simulink model "aocs_plant"  (R2025a)
settings: Solver=ode45  StartTime=0  StopTime=200  RelTol=1e-09  AbsTol=1e-10
undefined symbols (not defined in the file): AOCS, AOCS_Config, AOCS_EnvironmentConfig, AOCS_GNCConfig, AOCS_OrbitConfig, AOCS_SensorConfig, IAU, juliandate, propagateOnboardSgp4
libraries: aerolibtransform2 x8, simulink x8, matrix_library x5
(part 2 of 3)

== system aocs_plant/GNC/Onboard Reference Vectors/Reference Validity ==
  SunVector : Inport
  MagneticVector : Inport  Port=2
  MinimumNorm : Inport  Port=3
  OrbitValid : Inport  Port=4
  Enabled : Inport  Port=5
  Magnetic Exists : RelationalOperator  Operator=>  OutDataTypeStr=boolean  RndMeth=Simplest  InputSameDT=off
  Magnetic Norm Squared : DotProduct  OutDataTypeStr=Inherit: Inherit via internal rule
  Minimum Norm Squared : Product
  References Valid : Logic  Inputs=4  AllPortsSameDT=off  OutDataTypeStr=boolean
  Sun Exists : RelationalOperator  Operator=>  OutDataTypeStr=boolean  RndMeth=Simplest  InputSameDT=off
  Sun Norm Squared : DotProduct  OutDataTypeStr=Inherit: Inherit via internal rule
  To Double : DataTypeConversion  OutDataTypeStr=double  SaturateOnIntegerOverflow=off  RndMeth=Floor
  Valid : Outport
  wires:
  Minimum Norm Squared/1 -> Sun Exists/2, Magnetic Exists/2
  Sun Exists/1 -> References Valid/1
  Magnetic Exists/1 -> References Valid/2
  OrbitValid/1 -> References Valid/3
  Enabled/1 -> References Valid/4
  References Valid/1 -> To Double/1
  To Double/1 -> Valid/1
  SunVector/1 -> Sun Norm Squared/2, Sun Norm Squared/1
  MagneticVector/1 -> Magnetic Norm Squared/2, Magnetic Norm Squared/1
  MinimumNorm/1 -> Minimum Norm Squared/2, Minimum Norm Squared/1
  Sun Norm Squared/1 -> Sun Exists/1
  Magnetic Norm Squared/1 -> Magnetic Exists/1

== system aocs_plant/GNC/Onboard Reference Vectors/Sun Reference Model ==
  r_I_m : Inport
  EnvironmentContext : Inport  Port=2  OutDataTypeStr=Bus: EnvironmentContextBus
  MinimumVectorNorm : Inport  Port=3
  Julian Date : Sum
  Normalize Sun Vector : Subsystem
  Planetary Ephemeris : PlanetaryEphem  units=m,m/s  target=Sun  useDateRange=on  startDate=juliandate(2020, 1, 1, 0, 0, 0)  endDate=juliandate(2030, 1, 1, 0, 0, 0)  outputVelocity=off
  Seconds to Julian Days : Gain  Gain=1/86400
  Select Time Context : BusSelector  OutputSignals=epoch_tdb_jd,t_s
  Spacecraft to Sun Vector : Sum  Inputs=+-
  Sun Vector Column : Reshape  OutputDimensionality=Customize  OutputDimensions=[3 1]
  Unused Sun Distance : Terminator
  sun_I_unit : Outport
  wires:
  EnvironmentContext/1 -> Select Time Context/1
  Select Time Context/2 -> Seconds to Julian Days/1  "<t_s>"
  Select Time Context/1 -> Julian Date/1  "<epoch_tdb_jd>"
  Seconds to Julian Days/1 -> Julian Date/2
  Julian Date/1 -> Planetary Ephemeris/1
  Planetary Ephemeris/1 -> Sun Vector Column/1
  Sun Vector Column/1 -> Spacecraft to Sun Vector/1
  r_I_m/1 -> Spacecraft to Sun Vector/2
  Spacecraft to Sun Vector/1 -> Normalize Sun Vector/1(Vector)
  MinimumVectorNorm/1 -> Normalize Sun Vector/2(MinimumNorm)
  Normalize Sun Vector/1(UnitVector) -> sun_I_unit/1
  Normalize Sun Vector/2(VectorNorm) -> Unused Sun Distance/1

== system aocs_plant/GNC/TRIAD Initialization/CSS Freshness ==
  CurrentTime : Inport
  ReportValid : Inport  Port=2
  ReceiveTime : Inport  Port=3
  Enabled : Inport  Port=4
  MaxAge : Inport  Port=5
  Age Within Limit : RelationalOperator  Operator=<=  OutDataTypeStr=boolean  RndMeth=Simplest  InputSameDT=off
  Fresh : Logic  Inputs=3  AllPortsSameDT=off  OutDataTypeStr=boolean
  Half : Constant  Value=0.5
  Report Age : Sum  Inputs=+-
  Report Is Valid : RelationalOperator  Operator=>  OutDataTypeStr=boolean  RndMeth=Simplest  InputSameDT=off
  Subsystem Enabled : RelationalOperator  Operator=>  OutDataTypeStr=boolean  RndMeth=Simplest  InputSameDT=off
  To Double : DataTypeConversion  OutDataTypeStr=double  SaturateOnIntegerOverflow=off  RndMeth=Floor
  Current : Outport
  wires:
  CurrentTime/1 -> Report Age/1
  ReceiveTime/1 -> Report Age/2
  Report Age/1 -> Age Within Limit/1
  MaxAge/1 -> Age Within Limit/2
  ReportValid/1 -> Report Is Valid/1
  Half/1 -> Report Is Valid/2, Subsystem Enabled/2
  Enabled/1 -> Subsystem Enabled/1
  Age Within Limit/1 -> Fresh/1
  Report Is Valid/1 -> Fresh/2
  Subsystem Enabled/1 -> Fresh/3
  Fresh/1 -> To Double/1
  To Double/1 -> Current/1

== system aocs_plant/GNC/TRIAD Initialization/Magnetometer Freshness ==
  CurrentTime : Inport
  ReportValid : Inport  Port=2
  ReceiveTime : Inport  Port=3
  Enabled : Inport  Port=4
  MaxAge : Inport  Port=5
  Age Within Limit : RelationalOperator  Operator=<=  OutDataTypeStr=boolean  RndMeth=Simplest  InputSameDT=off
  Fresh : Logic  Inputs=3  AllPortsSameDT=off  OutDataTypeStr=boolean
  Half : Constant  Value=0.5
  Report Age : Sum  Inputs=+-
  Report Is Valid : RelationalOperator  Operator=>  OutDataTypeStr=boolean  RndMeth=Simplest  InputSameDT=off
  Subsystem Enabled : RelationalOperator  Operator=>  OutDataTypeStr=boolean  RndMeth=Simplest  InputSameDT=off
  To Double : DataTypeConversion  OutDataTypeStr=double  SaturateOnIntegerOverflow=off  RndMeth=Floor
  Current : Outport
  wires:
  CurrentTime/1 -> Report Age/1
  ReceiveTime/1 -> Report Age/2
  Report Age/1 -> Age Within Limit/1
  MaxAge/1 -> Age Within Limit/2
  ReportValid/1 -> Report Is Valid/1
  Half/1 -> Report Is Valid/2, Subsystem Enabled/2
  Enabled/1 -> Subsystem Enabled/1
  Age Within Limit/1 -> Fresh/1
  Report Is Valid/1 -> Fresh/2
  Subsystem Enabled/1 -> Fresh/3
  Fresh/1 -> To Double/1
  To Double/1 -> Current/1

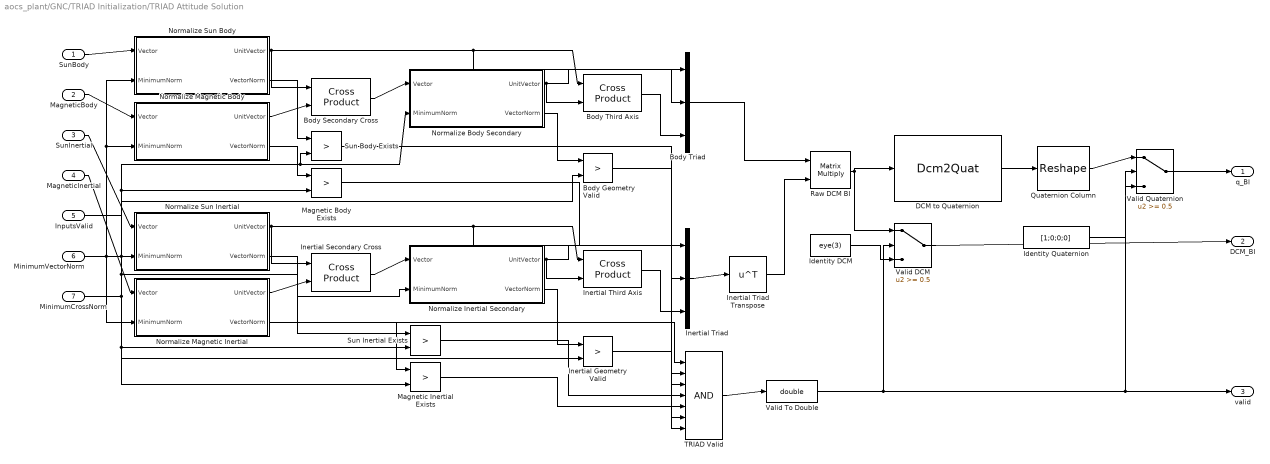
== system aocs_plant/GNC/TRIAD Initialization/TRIAD Attitude Solution ==
  SunBody : Inport
  MagneticBody : Inport  Port=2
  SunInertial : Inport  Port=3
  MagneticInertial : Inport  Port=4
  InputsValid : Inport  Port=5
  MinimumVectorNorm : Inport  Port=6
  MinimumCrossNorm : Inport  Port=7
  Body Geometry Valid : RelationalOperator  Operator=>  OutDataTypeStr=boolean  RndMeth=Simplest  InputSameDT=off
  Body Secondary Cross : matrix_library/Cross Product
  Body Third Axis : matrix_library/Cross Product
  Body Triad : Concatenate  NumInputs=3  Mode=Multidimensional array  ConcatenateDimension=2
  DCM to Quaternion : Dcm2Quat
  Identity DCM : Constant  Value=eye(3)
  Identity Quaternion : Constant  Value=[1;0;0;0]
  Inertial Geometry Valid : RelationalOperator  Operator=>  OutDataTypeStr=boolean  RndMeth=Simplest  InputSameDT=off
  Inertial Secondary Cross : matrix_library/Cross Product
  Inertial Third Axis : matrix_library/Cross Product
  Inertial Triad : Concatenate  NumInputs=3  Mode=Multidimensional array  ConcatenateDimension=2
  Inertial Triad Transpose : Math  Operator=transpose
  Magnetic Body Exists : RelationalOperator  Operator=>  OutDataTypeStr=boolean  RndMeth=Simplest  InputSameDT=off
  Magnetic Inertial Exists : RelationalOperator  Operator=>  OutDataTypeStr=boolean  RndMeth=Simplest  InputSameDT=off
  Normalize Body Secondary : Subsystem
  Normalize Inertial Secondary : Subsystem
  Normalize Magnetic Body : Subsystem
  Normalize Magnetic Inertial : Subsystem
  Normalize Sun Body : Subsystem
  Normalize Sun Inertial : Subsystem
  Quaternion Column : Reshape  OutputDimensionality=Customize  OutputDimensions=[4 1]
  Raw DCM BI : Product  Multiplication=Matrix(*)
  Sun Body Exists : RelationalOperator  Operator=>  OutDataTypeStr=boolean  RndMeth=Simplest  InputSameDT=off
  Sun Inertial Exists : RelationalOperator  Operator=>  OutDataTypeStr=boolean  RndMeth=Simplest  InputSameDT=off
  TRIAD Valid : Logic  Inputs=7  AllPortsSameDT=off  OutDataTypeStr=boolean
  Valid DCM : Switch  Threshold=0.5  SaturateOnIntegerOverflow=off  InputSameDT=off
  Valid Quaternion : Switch  Threshold=0.5  SaturateOnIntegerOverflow=off  InputSameDT=off
  Valid To Double : DataTypeConversion  OutDataTypeStr=double  SaturateOnIntegerOverflow=off  RndMeth=Floor
  q_BI : Outport
  DCM_BI : Outport  Port=2
  valid : Outport  Port=3
  wires:
  SunBody/1 -> Normalize Sun Body/1(Vector)
  MinimumVectorNorm/1 -> Sun Inertial Exists/2, Magnetic Inertial Exists/2, Normalize Inertial Secondary/2(MinimumNorm), Normalize Body Secondary/2(MinimumNorm), Sun Body Exists/2, Magnetic Body Exists/2, Normalize Sun Inertial/2(MinimumNorm), Normalize Sun Body/2(MinimumNorm), Normalize Magnetic Body/2(MinimumNorm), Normalize Magnetic Inertial/2(MinimumNorm)
  MagneticBody/1 -> Normalize Magnetic Body/1(Vector)
  SunInertial/1 -> Normalize Sun Inertial/1(Vector)
  MagneticInertial/1 -> Normalize Magnetic Inertial/1(Vector)
  Normalize Sun Body/1(UnitVector) -> Body Third Axis/1, Body Triad/1, Body Secondary Cross/1
  Normalize Magnetic Body/1(UnitVector) -> Body Secondary Cross/2
  Body Secondary Cross/1 -> Normalize Body Secondary/1(Vector)
  Normalize Body Secondary/1(UnitVector) -> Body Third Axis/2, Body Triad/2
  Body Third Axis/1 -> Body Triad/3
  Normalize Sun Inertial/1(UnitVector) -> Inertial Third Axis/1, Inertial Triad/1, Inertial Secondary Cross/1
  Normalize Magnetic Inertial/1(UnitVector) -> Inertial Secondary Cross/2
  Inertial Secondary Cross/1 -> Normalize Inertial Secondary/1(Vector)
  Normalize Inertial Secondary/1(UnitVector) -> Inertial Third Axis/2, Inertial Triad/2
  Inertial Third Axis/1 -> Inertial Triad/3
  Inertial Triad/1 -> Inertial Triad Transpose/1
  Body Triad/1 -> Raw DCM BI/1
  Inertial Triad Transpose/1 -> Raw DCM BI/2
  Raw DCM BI/1 -> DCM to Quaternion/1, Valid DCM/1
  DCM to Quaternion/1 -> Quaternion Column/1
  Normalize Sun Body/2(VectorNorm) -> Sun Body Exists/1
  Normalize Magnetic Body/2(VectorNorm) -> Magnetic Body Exists/1
  Normalize Sun Inertial/2(VectorNorm) -> Sun Inertial Exists/1
  Normalize Magnetic Inertial/2(VectorNorm) -> Magnetic Inertial Exists/1
  Normalize Body Secondary/2(VectorNorm) -> Body Geometry Valid/1
  MinimumCrossNorm/1 -> Body Geometry Valid/2, Inertial Geometry Valid/2
  Normalize Inertial Secondary/2(VectorNorm) -> Inertial Geometry Valid/1
  InputsValid/1 -> TRIAD Valid/1
  Sun Body Exists/1 -> TRIAD Valid/2
  Magnetic Body Exists/1 -> TRIAD Valid/3
  Sun Inertial Exists/1 -> TRIAD Valid/4
  Magnetic Inertial Exists/1 -> TRIAD Valid/5
  Body Geometry Valid/1 -> TRIAD Valid/6
  Inertial Geometry Valid/1 -> TRIAD Valid/7
  TRIAD Valid/1 -> Valid To Double/1
  Quaternion Column/1 -> Valid Quaternion/1
  Valid To Double/1 -> Valid Quaternion/2, valid/1, Valid DCM/2
  Identity Quaternion/1 -> Valid Quaternion/3
  Identity DCM/1 -> Valid DCM/3
  Valid Quaternion/1 -> q_BI/1
  Valid DCM/1 -> DCM_BI/1

== system aocs_plant/Sensors/GNSS/Fix Availability ==
  GnssConfig : Inport
  Acquisition Complete : RelationalOperator  OutDataTypeStr=boolean  RndMeth=Simplest  InputSameDT=off
  Configured Dropout : simulink/Logic and Bit Operations/Compare To Constant  relop===  const=2  OutDataTypeStr=boolean
  Dropout Uniform : UniformRandomNumber  Minimum=0  Seed=AOCS_SensorConfig.GNSS.dropout_seed  SampleTime=AOCS_SensorConfig.GNSS.sample_time_s
  Fix Available : Logic  Inputs=3  AllPortsSameDT=off  OutDataTypeStr=boolean
  No Configured Dropout : Logic  Operator=NOT  AllPortsSameDT=off  OutDataTypeStr=boolean
  No Random Dropout : Logic  Operator=NOT  AllPortsSameDT=off  OutDataTypeStr=boolean
  Random Dropout : RelationalOperator  Operator=<  OutDataTypeStr=boolean  RndMeth=Simplest  InputSameDT=off
  Select Availability Config : BusSelector  OutputSignals=mode_id,acquisition_time_s,dropout_probability_per_sample
  Simulation Time : Clock
  To Double : DataTypeConversion  OutDataTypeStr=double  SaturateOnIntegerOverflow=off  RndMeth=Floor
  fix_available : Outport
  wires:
  GnssConfig/1 -> Select Availability Config/1
  Simulation Time/1 -> Acquisition Complete/1
  Select Availability Config/2 -> Acquisition Complete/2  "<acquisition_time_s>"
  Dropout Uniform/1 -> Random Dropout/1
  Select Availability Config/3 -> Random Dropout/2  "<dropout_probability_per_sample>"
  Select Availability Config/1 -> Configured Dropout/1  "<mode_id>"
  Random Dropout/1 -> No Random Dropout/1
  Configured Dropout/1 -> No Configured Dropout/1
  Acquisition Complete/1 -> Fix Available/1
  No Random Dropout/1 -> Fix Available/2
  No Configured Dropout/1 -> Fix Available/3
  Fix Available/1 -> To Double/1
  To Double/1 -> fix_available/1  "fix_available"

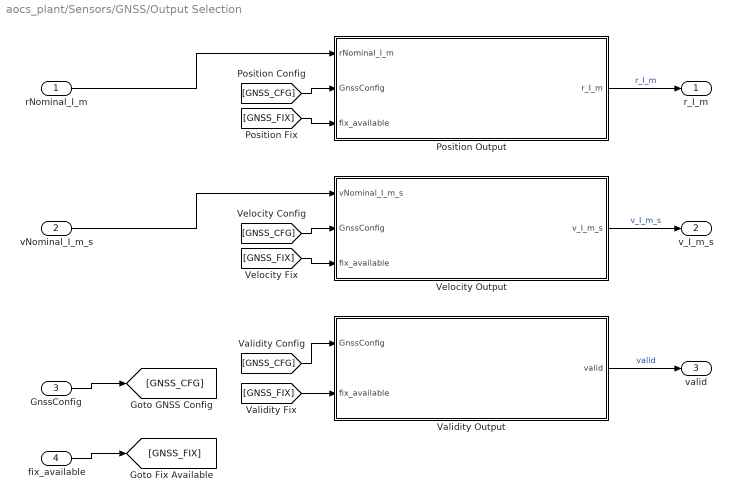
== system aocs_plant/Sensors/GNSS/Output Selection ==
  rNominal_I_m : Inport
  vNominal_I_m_s : Inport  Port=2
  GnssConfig : Inport  Port=3
  fix_available : Inport  Port=4
  Position Output : Subsystem
  Validity Output : Subsystem
  Velocity Output : Subsystem
  r_I_m : Outport
  v_I_m_s : Outport  Port=2
  valid : Outport  Port=3
  wires:
  GnssConfig/1 -> [GNSS_CFG]
  fix_available/1 -> [GNSS_FIX]
  rNominal_I_m/1 -> Position Output/1(rNominal_I_m)
  [GNSS_CFG] -> Position Output/2(GnssConfig)
  [GNSS_FIX] -> Position Output/3(fix_available)
  Position Output/1(r_I_m) -> r_I_m/1  "r_I_m"
  vNominal_I_m_s/1 -> Velocity Output/1(vNominal_I_m_s)
  [GNSS_CFG] -> Velocity Output/2(GnssConfig)
  [GNSS_FIX] -> Velocity Output/3(fix_available)
  Velocity Output/1(v_I_m_s) -> v_I_m_s/1  "v_I_m_s"
  [GNSS_CFG] -> Validity Output/1(GnssConfig)
  [GNSS_FIX] -> Validity Output/2(fix_available)
  Validity Output/1(valid) -> valid/1  "valid"

== system aocs_plant/Sensors/GNSS/PVT Error Model ==
  rTruth_I_m : Inport
  vTruth_I_m_s : Inport  Port=2
  Apply RTN Errors : MATLAB Function  TreatAsAtomicUnit=on
  Position Error RTN : Subsystem
  Velocity Error RTN : Subsystem
  rMeasured_I_m : Outport
  vMeasured_I_m_s : Outport  Port=2
  wires:
  rTruth_I_m/1 -> Apply RTN Errors/1(rTruth_I_m)
  vTruth_I_m_s/1 -> Apply RTN Errors/2(vTruth_I_m_s)
  Position Error RTN/1(positionError_RTN_m) -> Apply RTN Errors/3(positionError_RTN_m)
  Velocity Error RTN/1(velocityError_RTN_m_s) -> Apply RTN Errors/4(velocityError_RTN_m_s)
  Apply RTN Errors/1(rMeasured_I_m) -> rMeasured_I_m/1  "r_measured_I_m"
  Apply RTN Errors/2(vMeasured_I_m_s) -> vMeasured_I_m_s/1  "v_measured_I_m_s"

== system aocs_plant/Sensors/Gyro/Bias ==
  Add : Sum
  Gain : Gain  Gain=AOCS_SensorConfig.Gyro.bias_random_walk_step_std_rad_s
  Random Number : RandomNumber  Seed=AOCS_SensorConfig.Gyro.bias_seed  SampleTime=AOCS_SensorConfig.Gyro.gyro_sample_time_s
  Unit Delay : UnitDelay  InitialCondition=AOCS_SensorConfig.Gyro.bias_initial_rad_s  SampleTime=AOCS_SensorConfig.Gyro.gyro_sample_time_s  HasFrameUpgradeWarning=on
  bias_rad_s : Outport
  wires:
  Random Number/1 -> Gain/1
  Gain/1 -> Add/1
  Add/1 -> Unit Delay/1
  Unit Delay/1 -> Add/2, bias_rad_s/1

== system aocs_plant/Sensors/Magnetometer/Bias ==
  Add : Sum
  Gain : Gain  Gain=AOCS_SensorConfig.Magnetometer.bias_random_walk_step_std_T
  Random Number : RandomNumber  Seed=AOCS_SensorConfig.Magnetometer.bias_seed  SampleTime=AOCS_SensorConfig.Magnetometer.sample_time_s
  Unit Delay : UnitDelay  InitialCondition=AOCS_SensorConfig.Magnetometer.bias_initial_T  SampleTime=AOCS_SensorConfig.Magnetometer.sample_time_s  HasFrameUpgradeWarning=on
  bias_T : Outport
  wires:
  Unit Delay/1 -> bias_T/1, Add/2
  Add/1 -> Unit Delay/1
  Gain/1 -> Add/1
  Random Number/1 -> Gain/1

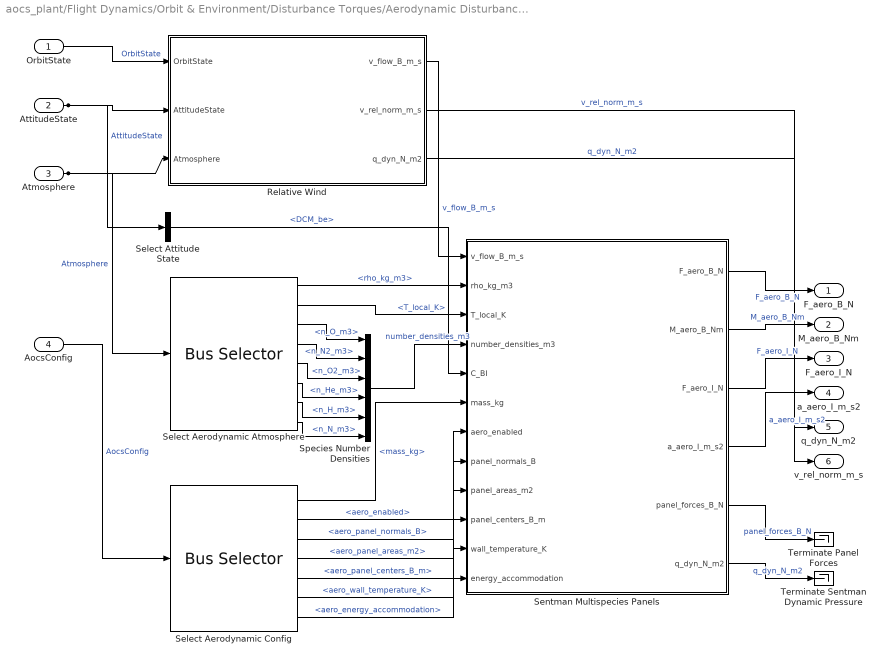
== system aocs_plant/Flight Dynamics/Orbit & Environment/Disturbance Torques/Aerodynamic Disturbance Path ==
  OrbitState : Inport
  AttitudeState : Inport  Port=2
  Atmosphere : Inport  Port=3
  AocsConfig : Inport  Port=4
  Relative Wind : Subsystem
  Select Aerodynamic Atmosphere : BusSelector  OutputSignals=rho_kg_m3,T_local_K,n_O_m3,n_N2_m3,n_O2_m3,n_He_m3,n_H_m3,n_N_m3
  Select Aerodynamic Config : BusSelector  OutputSignals=mass_kg,aero_enabled,aero_panel_normals_B,aero_panel_areas_m2,aero_panel_centers_B_m,aero_wall_temperature_K,aero_energy_accommodation
  Select Attitude State : BusSelector  OutputSignals=DCM_be
  Sentman Multispecies Panels : MATLAB Function  TreatAsAtomicUnit=on
  Species Number Densities : Mux  Inputs=6
  Terminate Panel Forces : Terminator
  Terminate Sentman Dynamic Pressure : Terminator
  F_aero_B_N : Outport
  M_aero_B_Nm : Outport  Port=2
  F_aero_I_N : Outport  Port=3
  a_aero_I_m_s2 : Outport  Port=4
  q_dyn_N_m2 : Outport  Port=5
  v_rel_norm_m_s : Outport  Port=6
  wires:
  OrbitState/1 -> Relative Wind/1(OrbitState)  "OrbitState"
  AttitudeState/1 -> Relative Wind/2(AttitudeState), Select Attitude State/1  "AttitudeState"
  Atmosphere/1 -> Relative Wind/3(Atmosphere), Select Aerodynamic Atmosphere/1  "Atmosphere"
  AocsConfig/1 -> Select Aerodynamic Config/1  "AocsConfig"
  Relative Wind/1(v_flow_B_m_s) -> Sentman Multispecies Panels/1(v_flow_B_m_s)  "v_flow_B_m_s"
  Select Aerodynamic Atmosphere/1 -> Sentman Multispecies Panels/2(rho_kg_m3)  "<rho_kg_m3>"
  Select Aerodynamic Atmosphere/2 -> Sentman Multispecies Panels/3(T_local_K)  "<T_local_K>"
  Select Aerodynamic Atmosphere/3 -> Species Number Densities/1  "<n_O_m3>"
  Select Aerodynamic Atmosphere/4 -> Species Number Densities/2  "<n_N2_m3>"
  Select Aerodynamic Atmosphere/5 -> Species Number Densities/3  "<n_O2_m3>"
  Select Aerodynamic Atmosphere/6 -> Species Number Densities/4  "<n_He_m3>"
  Select Aerodynamic Atmosphere/7 -> Species Number Densities/5  "<n_H_m3>"
  Select Aerodynamic Atmosphere/8 -> Species Number Densities/6  "<n_N_m3>"
  Species Number Densities/1 -> Sentman Multispecies Panels/4(number_densities_m3)  "number_densities_m3"
  Select Attitude State/1 -> Sentman Multispecies Panels/5(C_BI)  "<DCM_be>"
  Select Aerodynamic Config/1 -> Sentman Multispecies Panels/6(mass_kg)  "<mass_kg>"
  Select Aerodynamic Config/2 -> Sentman Multispecies Panels/7(aero_enabled)  "<aero_enabled>"
  Select Aerodynamic Config/3 -> Sentman Multispecies Panels/8(panel_normals_B)  "<aero_panel_normals_B>"
  Select Aerodynamic Config/4 -> Sentman Multispecies Panels/9(panel_areas_m2)  "<aero_panel_areas_m2>"
  Select Aerodynamic Config/5 -> Sentman Multispecies Panels/10(panel_centers_B_m)  "<aero_panel_centers_B_m>"
  Select Aerodynamic Config/6 -> Sentman Multispecies Panels/11(wall_temperature_K)  "<aero_wall_temperature_K>"
  Select Aerodynamic Config/7 -> Sentman Multispecies Panels/12(energy_accommodation)  "<aero_energy_accommodation>"
  Sentman Multispecies Panels/1(F_aero_B_N) -> F_aero_B_N/1  "F_aero_B_N"
  Sentman Multispecies Panels/2(M_aero_B_Nm) -> M_aero_B_Nm/1  "M_aero_B_Nm"
  Sentman Multispecies Panels/3(F_aero_I_N) -> F_aero_I_N/1  "F_aero_I_N"
  Sentman Multispecies Panels/4(a_aero_I_m_s2) -> a_aero_I_m_s2/1  "a_aero_I_m_s2"
  Relative Wind/3(q_dyn_N_m2) -> q_dyn_N_m2/1  "q_dyn_N_m2"
  Relative Wind/2(v_rel_norm_m_s) -> v_rel_norm_m_s/1  "v_rel_norm_m_s"
  Sentman Multispecies Panels/5(panel_forces_B_N) -> Terminate Panel Forces/1  "panel_forces_B_N"
  Sentman Multispecies Panels/6(q_dyn_N_m2) -> Terminate Sentman Dynamic Pressure/1  "q_dyn_N_m2"

== system aocs_plant/Flight Dynamics/Orbit & Environment/Disturbance Torques/Gravity Gradient Path ==
  OrbitState : Inport
  AttitudeState : Inport  Port=2
  AocsConfig : Inport  Port=3
  EnvironmentContext : Inport  Port=4
  EnvironmentConfig : Inport  Port=5
  Apply GG Enable : Product
  Gravity Gradient Torque : MATLAB Function  TreatAsAtomicUnit=on
  Select AOCS Config : BusSelector  OutputSignals=I_B
  Select Attitude State : BusSelector  OutputSignals=DCM_be
  Select Environment Config : BusSelector  OutputSignals=gravity_gradient_enabled
  Select Environment Context : BusSelector  OutputSignals=mu_m3_s2
  Select Orbit State : BusSelector  OutputSignals=r_I_m
  M_gg_B_Nm : Outport
  wires:
  OrbitState/1 -> Select Orbit State/1  "OrbitState"
  AttitudeState/1 -> Select Attitude State/1  "AttitudeState"
  AocsConfig/1 -> Select AOCS Config/1  "AocsConfig"
  EnvironmentContext/1 -> Select Environment Context/1  "EnvironmentContext"
  EnvironmentConfig/1 -> Select Environment Config/1  "EnvironmentConfig"
  Select Orbit State/1 -> Gravity Gradient Torque/1(r_I_m)  "<r_I_m>"
  Select Attitude State/1 -> Gravity Gradient Torque/2(DCM_be)  "<DCM_be>"
  Select AOCS Config/1 -> Gravity Gradient Torque/3(I_B)  "<I_B>"
  Select Environment Context/1 -> Apply GG Enable/1  "<mu_m3_s2>"
  Select Environment Config/1 -> Apply GG Enable/2  "<gravity_gradient_enabled>"
  Apply GG Enable/1 -> Gravity Gradient Torque/4(mu_m3_s2)  "mu_m3_s2"
  Gravity Gradient Torque/1(M_gg_B_Nm) -> M_gg_B_Nm/1  "M_gg_B_Nm"

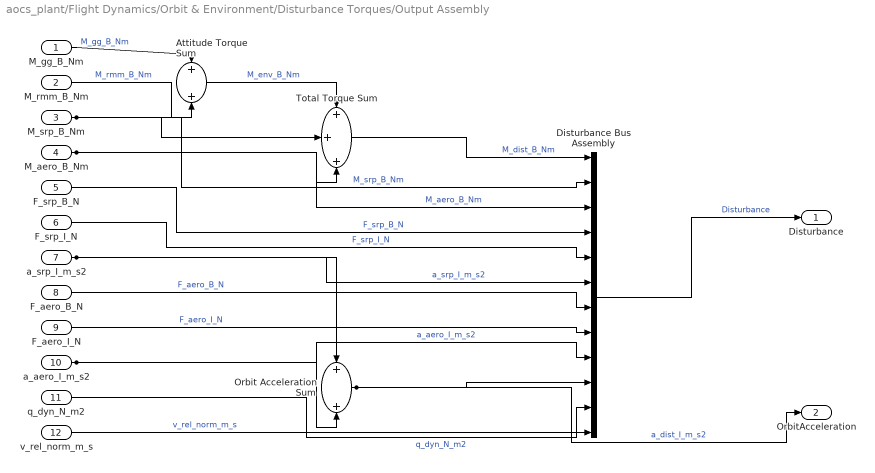
== system aocs_plant/Flight Dynamics/Orbit & Environment/Disturbance Torques/Output Assembly ==
  M_gg_B_Nm : Inport
  M_rmm_B_Nm : Inport  Port=2
  M_srp_B_Nm : Inport  Port=3
  M_aero_B_Nm : Inport  Port=4
  F_srp_B_N : Inport  Port=5
  F_srp_I_N : Inport  Port=6
  a_srp_I_m_s2 : Inport  Port=7
  F_aero_B_N : Inport  Port=8
  F_aero_I_N : Inport  Port=9
  a_aero_I_m_s2 : Inport  Port=10
  q_dyn_N_m2 : Inport  Port=11
  v_rel_norm_m_s : Inport  Port=12
  Attitude Torque Sum : Sum
  Disturbance Bus Assembly : BusCreator  Inputs=12  OutDataTypeStr=Bus: DisturbanceBus
  Orbit Acceleration Sum : Sum
  Total Torque Sum : Sum  Inputs=+++
  Disturbance : Outport
  OrbitAcceleration : Outport  Port=2
  wires:
  M_gg_B_Nm/1 -> Attitude Torque Sum/1  "M_gg_B_Nm"
  M_rmm_B_Nm/1 -> Attitude Torque Sum/2  "M_rmm_B_Nm"
  Attitude Torque Sum/1 -> Total Torque Sum/1  "M_env_B_Nm"
  M_srp_B_Nm/1 -> Total Torque Sum/2, Disturbance Bus Assembly/2  "M_srp_B_Nm"
  M_aero_B_Nm/1 -> Total Torque Sum/3, Disturbance Bus Assembly/3  "M_aero_B_Nm"
  a_srp_I_m_s2/1 -> Orbit Acceleration Sum/1, Disturbance Bus Assembly/6  "a_srp_I_m_s2"
  a_aero_I_m_s2/1 -> Orbit Acceleration Sum/2, Disturbance Bus Assembly/9  "a_aero_I_m_s2"
  Total Torque Sum/1 -> Disturbance Bus Assembly/1  "M_dist_B_Nm"
  F_srp_B_N/1 -> Disturbance Bus Assembly/4  "F_srp_B_N"
  F_srp_I_N/1 -> Disturbance Bus Assembly/5  "F_srp_I_N"
  F_aero_B_N/1 -> Disturbance Bus Assembly/7  "F_aero_B_N"
  F_aero_I_N/1 -> Disturbance Bus Assembly/8  "F_aero_I_N"
  Orbit Acceleration Sum/1 -> Disturbance Bus Assembly/10, OrbitAcceleration/1  "a_dist_I_m_s2"
  q_dyn_N_m2/1 -> Disturbance Bus Assembly/11  "q_dyn_N_m2"
  v_rel_norm_m_s/1 -> Disturbance Bus Assembly/12  "v_rel_norm_m_s"
  Disturbance Bus Assembly/1 -> Disturbance/1  "Disturbance"

== system aocs_plant/Flight Dynamics/Orbit & Environment/Disturbance Torques/Residual Magnetic Path ==
  EnvironmentConfig : Inport
  MagneticField : Inport  Port=2
  Apply RMM Enable : Product
  Cross Product : matrix_library/Cross Product
  Select Environment Config : BusSelector  OutputSignals=m_res_B_A_m2,rmm_enabled
  Select Magnetic Field : BusSelector  OutputSignals=B_B_T
  M_rmm_B_Nm : Outport
  wires:
  EnvironmentConfig/1 -> Select Environment Config/1  "EnvironmentConfig"
  MagneticField/1 -> Select Magnetic Field/1  "MagneticField"
  Select Environment Config/1 -> Apply RMM Enable/1  "<m_res_B_A_m2>"
  Select Environment Config/2 -> Apply RMM Enable/2  "<rmm_enabled>"
  Apply RMM Enable/1 -> Cross Product/1  "m_res_B_A_m2"
  Select Magnetic Field/1 -> Cross Product/2  "<B_B_T>"
  Cross Product/1 -> M_rmm_B_Nm/1  "M_rmm_B_Nm"

== system aocs_plant/Flight Dynamics/Orbit & Environment/Disturbance Torques/SRP Disturbance Path ==
  SRP : Inport
  AttitudeState : Inport  Port=2
  AocsConfig : Inport  Port=3
  SRP Inertial Acceleration : MATLAB Function  TreatAsAtomicUnit=on
  Select Attitude State : BusSelector  OutputSignals=DCM_be
  Select Mass : BusSelector  OutputSignals=mass_kg
  Select SRP : BusSelector  OutputSignals=M_srp_B_Nm,F_srp_B_N
  M_srp_B_Nm : Outport
  F_srp_B_N : Outport  Port=2
  F_srp_I_N : Outport  Port=3
  a_srp_I_m_s2 : Outport  Port=4
  wires:
  SRP/1 -> Select SRP/1  "SRP"
  AttitudeState/1 -> Select Attitude State/1  "AttitudeState"
  AocsConfig/1 -> Select Mass/1  "AocsConfig"
  Select SRP/1 -> M_srp_B_Nm/1  "<M_srp_B_Nm>"
  Select SRP/2 -> SRP Inertial Acceleration/1(F_srp_B_N), F_srp_B_N/1  "<F_srp_B_N>"
  Select Attitude State/1 -> SRP Inertial Acceleration/2(C_BI)  "<DCM_be>"
  Select Mass/1 -> SRP Inertial Acceleration/3(mass_kg)  "<mass_kg>"
  SRP Inertial Acceleration/1(F_srp_I_N) -> F_srp_I_N/1  "F_srp_I_N"
  SRP Inertial Acceleration/2(a_srp_I_m_s2) -> a_srp_I_m_s2/1  "a_srp_I_m_s2"

== system aocs_plant/Flight Dynamics/Orbit & Environment/Environment Products/Atmosphere Products ==
  EnvironmentConfig : Inport  OutDataTypeStr=Bus: EnvironmentConfigBus
  OrbitState : Inport  Port=2  OutDataTypeStr=Bus: OrbitStateBus
  EnvironmentContext : Inport  Port=3  OutDataTypeStr=Bus: EnvironmentContextBus
  Atmosphere Model : Subsystem
  Frame Transformations : Subsystem
  Terminate C_ECEF_ECI : Terminator
  Terminate v_ECEF_m_s : Terminator
  Atmosphere : Outport  OutDataTypeStr=Bus: AtmosphereBus
  wires:
  OrbitState/1 -> Frame Transformations/1(In1), Atmosphere Model/2(OrbitState)
  EnvironmentContext/1 -> Frame Transformations/2(In2), Atmosphere Model/4(EnvironmentContext)
  EnvironmentConfig/1 -> Atmosphere Model/1(EnvironmentConfig)
  Frame Transformations/1(lla) -> Atmosphere Model/3(lla)
  Frame Transformations/2(v_ECEF_m_s) -> Terminate v_ECEF_m_s/1
  Frame Transformations/3(C_ECEF_ECI) -> Terminate C_ECEF_ECI/1
  Atmosphere Model/1(Atmosphere) -> Atmosphere/1

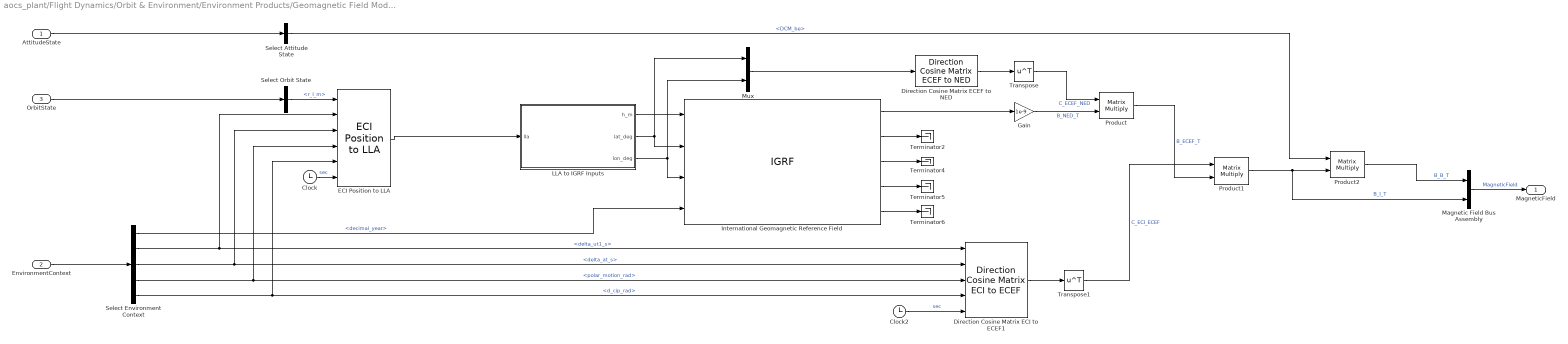
== system aocs_plant/Flight Dynamics/Orbit & Environment/Environment Products/Geomagnetic Field Model ==
  AttitudeState : Inport
  EnvironmentContext : Inport  Port=2
  OrbitState : Inport  Port=3
  Clock : Clock
  Clock2 : Clock
  Direction Cosine Matrix ECEF to NED : aerolibtransform2/Direction Cosine Matrix ECEF to NED
  Direction Cosine Matrix ECI to ECEF1 : aerolibtransform2/Direction Cosine Matrix ECI to ECEF  red=IAU-2000/2006  year=2026  month=January  day=1  hour=0  min=0  sec=0  deltaT=Sec  errorflag=Error  extraparamflag=on
      settings: AttributesFormatString=%<red>
  ECI Position to LLA : aerolibtransform2/ECI Position to LLA  red=IAU-2000/2006  year=2026  month=January  day=1  hour=0  min=0  sec=0  deltaT=Sec  errorflag=Error  extraparamflag=on  eunits=Metric (MKS)  earthmodel=WGS84  flat=1/298.257223563  eqradius=6378137
      settings: AttributesFormatString=%<red>
  Gain : Gain  Gain=1e-9
  International Geomagnetic Reference Field : IGRF  month=January  day=1  sv_out=off
      settings: AttributesFormatString=%<generation>
  LLA to IGRF Inputs : MATLAB Function  TreatAsAtomicUnit=on
  Magnetic Field Bus Assembly : BusCreator  Inputs=2  OutDataTypeStr=Bus: MagneticFieldBus
  Mux : Mux  Inputs=2
  Product : Product  Multiplication=Matrix(*)
  Product1 : Product  Multiplication=Matrix(*)
  Product2 : Product  Multiplication=Matrix(*)
  Select Attitude State : BusSelector  OutputSignals=DCM_be
  Select Environment Context : BusSelector  OutputSignals=decimal_year,delta_ut1_s,delta_at_s,polar_motion_rad,d_cip_rad
  Select Orbit State : BusSelector  OutputSignals=r_I_m
  Terminator{2,4..6} (4 alike) : Terminator
  Transpose : Math  Operator=transpose
  Transpose1 : Math  Operator=transpose
  MagneticField : Outport
  wires:
  Product2/1 -> Magnetic Field Bus Assembly/1  "B_B_T"
  Product1/1 -> Magnetic Field Bus Assembly/2, Product2/2  "B_I_T"
  Transpose1/1 -> Product1/1  "C_ECI_ECEF"
  Product/1 -> Product1/2  "B_ECEF_T"
  Direction Cosine Matrix ECI to ECEF1/1 -> Transpose1/1
  Transpose/1 -> Product/1  "C_ECEF_NED"
  Gain/1 -> Product/2  "B_NED_T"
  Direction Cosine Matrix ECEF to NED/1 -> Transpose/1
  International Geomagnetic Reference Field/2 -> Terminator2/1
  International Geomagnetic Reference Field/1 -> Gain/1
  Mux/1 -> Direction Cosine Matrix ECEF to NED/1
  International Geomagnetic Reference Field/5 -> Terminator6/1
  LLA to IGRF Inputs/2(lat_deg) -> International Geomagnetic Reference Field/2, Mux/1
  International Geomagnetic Reference Field/4 -> Terminator5/1
  LLA to IGRF Inputs/1(h_m) -> International Geomagnetic Reference Field/1
  LLA to IGRF Inputs/3(lon_deg) -> International Geomagnetic Reference Field/3, Mux/2
  International Geomagnetic Reference Field/3 -> Terminator4/1
  ECI Position to LLA/1 -> LLA to IGRF Inputs/1(lla)
  AttitudeState/1 -> Select Attitude State/1
  Select Attitude State/1 -> Product2/1  "<DCM_be>"
  OrbitState/1 -> Select Orbit State/1
  Select Orbit State/1 -> ECI Position to LLA/1  "<r_I_m>"
  EnvironmentContext/1 -> Select Environment Context/1
  Select Environment Context/1 -> International Geomagnetic Reference Field/4  "<decimal_year>"
  Magnetic Field Bus Assembly/1 -> MagneticField/1  "MagneticField"
  Select Environment Context/5 -> ECI Position to LLA/5, Direction Cosine Matrix ECI to ECEF1/4  "<d_cip_rad>"
  Clock/1 -> ECI Position to LLA/6  "sec"
  Clock2/1 -> Direction Cosine Matrix ECI to ECEF1/5  "sec"
  Select Environment Context/4 -> ECI Position to LLA/4, Direction Cosine Matrix ECI to ECEF1/3  "<polar_motion_rad>"
  Select Environment Context/2 -> Direction Cosine Matrix ECI to ECEF1/1, ECI Position to LLA/2  "<delta_ut1_s>"
  Select Environment Context/3 -> ECI Position to LLA/3, Direction Cosine Matrix ECI to ECEF1/2  "<delta_at_s>"

== system aocs_plant/Flight Dynamics/Orbit & Environment/Environment Products/Illumination Model ==
  OrbitState : Inport
  EnvironmentConfig : Inport  Port=2
  Sun : Inport  Port=3
  Eclipse Disabled Visibility : Constant  Value=1.0
  Eclipse Enable Switch : Switch  Threshold=0.5  SaturateOnIntegerOverflow=off  InputSameDT=off
  Eclipse Shadow Model (Dual Cone) : EclipseShadowModel  outputShadowRegion=on  startDate=juliandate(2026, 1, 1, 0, 0, 0)  customRadius=6378137  ephemerisStartDate=juliandate(2020, 1, 1, 0, 0, 0)  ephemerisEndDate=juliandate(2030, 1, 1, 0, 0, 0)
  Illumination Bus Assembly : BusCreator  Inputs=3  OutDataTypeStr=Bus: IlluminationBus
  Select Environment Config : BusSelector  OutputSignals=eclipse_enabled
  Select Orbit State : BusSelector  OutputSignals=r_I_m
  Select Sun : BusSelector  OutputSignals=solar_flux_W_m2
  Solar Flux Shadowing : Product
  Terminator : Terminator
  Terminator1 : Terminator
  Illumination : Outport
  wires:
  Eclipse Shadow Model (Dual Cone)/2 -> Terminator/1
  Eclipse Shadow Model (Dual Cone)/3 -> Terminator1/1
  Eclipse Shadow Model (Dual Cone)/1 -> Illumination Bus Assembly/1, Eclipse Enable Switch/1  "eclipse_fraction"
  OrbitState/1 -> Select Orbit State/1
  Select Orbit State/1 -> Eclipse Shadow Model (Dual Cone)/1  "<r_I_m>"
  EnvironmentConfig/1 -> Select Environment Config/1
  Select Environment Config/1 -> Eclipse Enable Switch/2  "<eclipse_enabled>"
  Eclipse Disabled Visibility/1 -> Eclipse Enable Switch/3
  Sun/1 -> Select Sun/1
  Select Sun/1 -> Solar Flux Shadowing/1  "<solar_flux_W_m2>"
  Eclipse Enable Switch/1 -> Solar Flux Shadowing/2, Illumination Bus Assembly/2  "sun_visibility"
  Solar Flux Shadowing/1 -> Illumination Bus Assembly/3  "solar_flux_shadowed_W_m2"
  Illumination Bus Assembly/1 -> Illumination/1  "Illumination"

== system aocs_plant/Flight Dynamics/Orbit & Environment/Environment Products/Solar Radiation Pressure ==
  Illumination : Inport
  Sun : Inport  Port=2
  MATLAB Function : MATLAB Function  TreatAsAtomicUnit=on
  SRP Bus Assembly : BusCreator  Inputs=3  OutDataTypeStr=Bus: SrpBus
  Select Illumination : BusSelector  OutputSignals=solar_flux_shadowed_W_m2
  Select Sun : BusSelector  OutputSignals=sun_B_unit
  srp_area_ref_m2 : Constant  Value=AOCS.EnvironmentConfig.srp_area_ref_m2  VectorParams1D=off  OutDataTypeStr=double
  srp_center_of_pressure_B_m : Constant  Value=AOCS.EnvironmentConfig.srp_center_of_pressure_B_m  VectorParams1D=off  OutDataTypeStr=double
  srp_coefficient_reflectivity : Constant  Value=AOCS.EnvironmentConfig.srp_coefficient_reflectivity  VectorParams1D=off  OutDataTypeStr=double
  srp_enabled : Constant  Value=AOCS.EnvironmentConfig.srp_enabled  VectorParams1D=off  OutDataTypeStr=double
  SRP : Outport
  wires:
  srp_enabled/1 -> MATLAB Function/3(srp_enabled)
  srp_area_ref_m2/1 -> MATLAB Function/4(srp_area_ref_m2)
  srp_coefficient_reflectivity/1 -> MATLAB Function/5(srp_coefficient_reflectivity)
  srp_center_of_pressure_B_m/1 -> MATLAB Function/6(srp_center_of_pressure_B_m)
  MATLAB Function/2(F_srp_B_N) -> SRP Bus Assembly/2  "F_srp_B_N"
  MATLAB Function/3(P_srp_N_m2) -> SRP Bus Assembly/3  "P_srp_N_m2"
  Sun/1 -> Select Sun/1  "Sun"
  Select Sun/1 -> MATLAB Function/1(sun_B_unit)  "<sun_B_unit>"
  Illumination/1 -> Select Illumination/1  "Illumination"
  Select Illumination/1 -> MATLAB Function/2(solar_flux_shadowed_W_m2)  "<solar_flux_shadowed_W_m2>"
  SRP Bus Assembly/1 -> SRP/1  "SRP"
  MATLAB Function/1(M_srp_B_Nm) -> SRP Bus Assembly/1  "M_srp_B_Nm"

== system aocs_plant/Flight Dynamics/Orbit & Environment/Environment Products/Sun Products ==
  EnvironmentConfig : Inport
  OrbitState : Inport  Port=2
  AttitudeState : Inport  Port=3
  EnvironmentContext : Inport  Port=4
  "  " : BusSelector  OutputSignals=solar_constant_W_m2
  Bus Selector : BusSelector  OutputSignals=r_I_m
  Bus Selector1 : BusSelector  OutputSignals=DCM_be
  Julian Date : Sum
  Planetary Ephemeris : PlanetaryEphem  units=m,m/s  target=Sun  useDateRange=on  startDate=juliandate(2020, 1, 1, 0, 0, 0)  endDate=juliandate(2030, 1, 1, 0, 0, 0)  outputVelocity=off
  Seconds to Julian Days : Gain  Gain=1/86400
  Select Environment Context : BusSelector  OutputSignals=epoch_tdb_jd,t_s
  Sun Bus Assembly : BusCreator  Inputs=5  OutDataTypeStr=Bus: SunBus
  Sun Geometry : MATLAB Function  TreatAsAtomicUnit=on
  Sun Vector Column : Reshape  OutputDimensionality=Customize  OutputDimensions=[3 1]
  Sun : Outport
  wires:
  EnvironmentContext/1 -> Select Environment Context/1
  Seconds to Julian Days/1 -> Julian Date/2
  Julian Date/1 -> Planetary Ephemeris/1
  Sun Geometry/1(sun_B_unit) -> Sun Bus Assembly/1  "sun_B_unit"
  Sun Geometry/2(sun_I_unit) -> Sun Bus Assembly/2  "sun_I_unit"
  Sun Geometry/3(r_sun_I_m) -> Sun Bus Assembly/3  "r_sun_I_m"
  Sun Geometry/4(sun_distance_m) -> Sun Bus Assembly/4  "sun_distance_m"
  Sun Geometry/5(solar_flux_W_m2) -> Sun Bus Assembly/5  "solar_flux_W_m2"
  Planetary Ephemeris/1 -> Sun Vector Column/1
  Sun Vector Column/1 -> Sun Geometry/1(r_sun_I_m_ephem)
  Select Environment Context/2 -> Seconds to Julian Days/1  "<t_s>"
  Select Environment Context/1 -> Julian Date/1  "<epoch_tdb_jd>"
  EnvironmentConfig/1 -> "  "/1
  "  "/1 -> Sun Geometry/2(solar_constant_W_m2)  "<solar_constant_W_m2>"
  OrbitState/1 -> Bus Selector/1
  Bus Selector/1 -> Sun Geometry/3(r_I_m)  "<r_I_m>"
  AttitudeState/1 -> Bus Selector1/1
  Bus Selector1/1 -> Sun Geometry/4(DCM_be)  "<DCM_be>"
  Sun Bus Assembly/1 -> Sun/1  "Sun"

== system aocs_plant/Flight Dynamics/Orbit & Environment/Orbit Propagator & Time/Orbit State ==
  OrbitAcceleration : Inport
  Orbit Propagator : Subsystem
  OrbitState : Outport
  wires:
  Orbit Propagator/1(OrbitState) -> OrbitState/1
  OrbitAcceleration/1 -> Orbit Propagator/1(OrbitAcceleration)

== system aocs_plant/Flight Dynamics/Orbit & Environment/Orbit Propagator & Time/Orbit and Time Context ==
  In1 : Inport
  Clock1 : Clock
  Delta AT : Constant  Value=AOCS.Environment.EarthOrientation.DeltaAT_s  OutDataTypeStr=double
  Delta CIP : Constant  Value=AOCS.Environment.EarthOrientation.DCIP_rad  OutDataTypeStr=double
  Delta UT1 : Constant  Value=AOCS.Environment.EarthOrientation.DeltaUT1_s  OutDataTypeStr=double
  Environment Context Bus Assembly : BusCreator  Inputs=9  OutDataTypeStr=Bus: EnvironmentContextBus
  MATLAB Function : MATLAB Function  TreatAsAtomicUnit=on
  Polar Motion : Constant  Value=AOCS.Environment.EarthOrientation.PolarMotion_rad  OutDataTypeStr=double
  Select Orbit Config : BusSelector  OutputSignals=epoch_utc,mu_m3_s2,epoch_tdb_jd
  EnvironmentContext : Outport
  wires:
  Select Orbit Config/2 -> Environment Context Bus Assembly/2  "<mu_m3_s2>"
  MATLAB Function/1(dyear) -> Environment Context Bus Assembly/1  "decimal_year"
  In1/1 -> Select Orbit Config/1
  Clock1/1 -> Environment Context Bus Assembly/4, MATLAB Function/2(t_s)  "t_s"
  Select Orbit Config/3 -> Environment Context Bus Assembly/5  "<epoch_tdb_jd>"
  Environment Context Bus Assembly/1 -> EnvironmentContext/1  "EnvironmentContext"
  Select Orbit Config/1 -> MATLAB Function/1(epoch_utc), Environment Context Bus Assembly/3  "<epoch_utc>"
  Delta AT/1 -> Environment Context Bus Assembly/6  "delta_at_s"
  Delta UT1/1 -> Environment Context Bus Assembly/7  "delta_ut1_s"
  Polar Motion/1 -> Environment Context Bus Assembly/8  "polar_motion_rad"
  Delta CIP/1 -> Environment Context Bus Assembly/9  "d_cip_rad"

== system aocs_plant/GNC/Onboard Reference Vectors/Sun Reference Model/Normalize Sun Vector ==
  Vector : Inport
  MinimumNorm : Inport  Port=2
  Norm : Math  Operator=sqrt
  Norm Squared : DotProduct  OutDataTypeStr=Inherit: Inherit via internal rule
  Normalize : Product  Inputs=*/
  Safe Norm : MinMax  Function=max  Inputs=2
  UnitVector : Outport
  VectorNorm : Outport  Port=2
  wires:
  Vector/1 -> Normalize/1, Norm Squared/1, Norm Squared/2
  Norm Squared/1 -> Norm/1
  Norm/1 -> VectorNorm/1, Safe Norm/1
  MinimumNorm/1 -> Safe Norm/2
  Safe Norm/1 -> Normalize/2
  Normalize/1 -> UnitVector/1

== system aocs_plant/GNC/TRIAD Initialization/TRIAD Attitude Solution/Normalize Body Secondary ==
  Vector : Inport
  MinimumNorm : Inport  Port=2
  Norm : Math  Operator=sqrt
  Norm Squared : DotProduct  OutDataTypeStr=Inherit: Inherit via internal rule
  Normalize : Product  Inputs=*/
  Safe Norm : MinMax  Function=max  Inputs=2
  UnitVector : Outport
  VectorNorm : Outport  Port=2
  wires:
  Vector/1 -> Norm Squared/1, Norm Squared/2, Normalize/1
  Norm Squared/1 -> Norm/1
  Norm/1 -> Safe Norm/1, VectorNorm/1
  MinimumNorm/1 -> Safe Norm/2
  Safe Norm/1 -> Normalize/2
  Normalize/1 -> UnitVector/1

== system aocs_plant/GNC/TRIAD Initialization/TRIAD Attitude Solution/Normalize Inertial Secondary ==
  Vector : Inport
  MinimumNorm : Inport  Port=2
  Norm : Math  Operator=sqrt
  Norm Squared : DotProduct  OutDataTypeStr=Inherit: Inherit via internal rule
  Normalize : Product  Inputs=*/
  Safe Norm : MinMax  Function=max  Inputs=2
  UnitVector : Outport
  VectorNorm : Outport  Port=2
  wires:
  Vector/1 -> Norm Squared/1, Norm Squared/2, Normalize/1
  Norm Squared/1 -> Norm/1
  Norm/1 -> Safe Norm/1, VectorNorm/1
  MinimumNorm/1 -> Safe Norm/2
  Safe Norm/1 -> Normalize/2
  Normalize/1 -> UnitVector/1

== system aocs_plant/GNC/TRIAD Initialization/TRIAD Attitude Solution/Normalize Magnetic Body ==
  Vector : Inport
  MinimumNorm : Inport  Port=2
  Norm : Math  Operator=sqrt
  Norm Squared : DotProduct  OutDataTypeStr=Inherit: Inherit via internal rule
  Normalize : Product  Inputs=*/
  Safe Norm : MinMax  Function=max  Inputs=2
  UnitVector : Outport
  VectorNorm : Outport  Port=2
  wires:
  Vector/1 -> Norm Squared/1, Norm Squared/2, Normalize/1
  Norm Squared/1 -> Norm/1
  Norm/1 -> Safe Norm/1, VectorNorm/1
  MinimumNorm/1 -> Safe Norm/2
  Safe Norm/1 -> Normalize/2
  Normalize/1 -> UnitVector/1

== system aocs_plant/GNC/TRIAD Initialization/TRIAD Attitude Solution/Normalize Magnetic Inertial ==
  Vector : Inport
  MinimumNorm : Inport  Port=2
  Norm : Math  Operator=sqrt
  Norm Squared : DotProduct  OutDataTypeStr=Inherit: Inherit via internal rule
  Normalize : Product  Inputs=*/
  Safe Norm : MinMax  Function=max  Inputs=2
  UnitVector : Outport
  VectorNorm : Outport  Port=2
  wires:
  Vector/1 -> Norm Squared/1, Norm Squared/2, Normalize/1
  Norm Squared/1 -> Norm/1
  Norm/1 -> Safe Norm/1, VectorNorm/1
  MinimumNorm/1 -> Safe Norm/2
  Safe Norm/1 -> Normalize/2
  Normalize/1 -> UnitVector/1

== system aocs_plant/GNC/TRIAD Initialization/TRIAD Attitude Solution/Normalize Sun Body ==
  Vector : Inport
  MinimumNorm : Inport  Port=2
  Norm : Math  Operator=sqrt
  Norm Squared : DotProduct  OutDataTypeStr=Inherit: Inherit via internal rule
  Normalize : Product  Inputs=*/
  Safe Norm : MinMax  Function=max  Inputs=2
  UnitVector : Outport
  VectorNorm : Outport  Port=2
  wires:
  Vector/1 -> Norm Squared/1, Norm Squared/2, Normalize/1
  Norm Squared/1 -> Norm/1
  Norm/1 -> Safe Norm/1, VectorNorm/1
  MinimumNorm/1 -> Safe Norm/2
  Safe Norm/1 -> Normalize/2
  Normalize/1 -> UnitVector/1

== system aocs_plant/GNC/TRIAD Initialization/TRIAD Attitude Solution/Normalize Sun Inertial ==
  Vector : Inport
  MinimumNorm : Inport  Port=2
  Norm : Math  Operator=sqrt
  Norm Squared : DotProduct  OutDataTypeStr=Inherit: Inherit via internal rule
  Normalize : Product  Inputs=*/
  Safe Norm : MinMax  Function=max  Inputs=2
  UnitVector : Outport
  VectorNorm : Outport  Port=2
  wires:
  Vector/1 -> Norm Squared/1, Norm Squared/2, Normalize/1
  Norm Squared/1 -> Norm/1
  Norm/1 -> Safe Norm/1, VectorNorm/1
  MinimumNorm/1 -> Safe Norm/2
  Safe Norm/1 -> Normalize/2
  Normalize/1 -> UnitVector/1

== system aocs_plant/Sensors/GNSS/Output Selection/Position Output ==
  rNominal_I_m : Inport
  GnssConfig : Inport  Port=2
  fix_available : Inport  Port=3
  Disabled Output : Constant  Value=zeros(3,1)
  Is Failure : simulink/Logic and Bit Operations/Compare To Constant  relop===  const=3  OutDataTypeStr=boolean
  No Fix Output : Constant  Value=zeros(3,1)
  Select Enabled : Switch  Criteria=u2 > Threshold  Threshold=0.5  SaturateOnIntegerOverflow=off  InputSameDT=off
  Select Failure : Switch  Criteria=u2 > Threshold  Threshold=0.5  SaturateOnIntegerOverflow=off  InputSameDT=off
  Select Fix : Switch  Criteria=u2 > Threshold  Threshold=0.5  SaturateOnIntegerOverflow=off  InputSameDT=off
  Select GNSS Config : BusSelector  OutputSignals=enabled,mode_id,failure_r_I_m
  r_I_m : Outport
  wires:
  rNominal_I_m/1 -> Select Fix/1
  fix_available/1 -> Select Fix/2
  No Fix Output/1 -> Select Fix/3
  [FAIL_VALUE] -> Select Failure/1
  [IS_FAILURE] -> Select Failure/2
  Select Fix/1 -> Select Failure/3
  Select Failure/1 -> Select Enabled/1
  [ENABLED] -> Select Enabled/2
  Disabled Output/1 -> Select Enabled/3
  Select Enabled/1 -> r_I_m/1  "r_I_m"
  GnssConfig/1 -> Select GNSS Config/1
  Select GNSS Config/1 -> [ENABLED]  "<enabled>"
  Select GNSS Config/2 -> Is Failure/1  "<mode_id>"
  Is Failure/1 -> [IS_FAILURE]
  Select GNSS Config/3 -> [FAIL_VALUE]  "<failure_r_I_m>"

== system aocs_plant/Sensors/GNSS/Output Selection/Validity Output ==
  GnssConfig : Inport
  fix_available : Inport  Port=2
  Disabled Invalid : Constant  Value=0
  Is Failure : simulink/Logic and Bit Operations/Compare To Constant  relop===  const=3  OutDataTypeStr=boolean
  No Fix Invalid : Constant  Value=0
  Nominal Valid : Constant
  Select Enabled : Switch  Criteria=u2 > Threshold  Threshold=0.5  SaturateOnIntegerOverflow=off  InputSameDT=off
  Select Failure : Switch  Criteria=u2 > Threshold  Threshold=0.5  SaturateOnIntegerOverflow=off  InputSameDT=off
  Select Fix : Switch  Criteria=u2 > Threshold  Threshold=0.5  SaturateOnIntegerOverflow=off  InputSameDT=off
  Select GNSS Config : BusSelector  OutputSignals=enabled,mode_id,failure_valid
  valid : Outport
  wires:
  Nominal Valid/1 -> Select Fix/1
  fix_available/1 -> Select Fix/2
  No Fix Invalid/1 -> Select Fix/3
  [FAIL_VALUE] -> Select Failure/1
  [IS_FAILURE] -> Select Failure/2
  Select Fix/1 -> Select Failure/3
  Select Failure/1 -> Select Enabled/1
  [ENABLED] -> Select Enabled/2
  Disabled Invalid/1 -> Select Enabled/3
  Select Enabled/1 -> valid/1  "valid"
  GnssConfig/1 -> Select GNSS Config/1
  Select GNSS Config/1 -> [ENABLED]  "<enabled>"
  Select GNSS Config/2 -> Is Failure/1  "<mode_id>"
  Is Failure/1 -> [IS_FAILURE]
  Select GNSS Config/3 -> [FAIL_VALUE]  "<failure_valid>"

== system aocs_plant/Sensors/GNSS/Output Selection/Velocity Output ==
  vNominal_I_m_s : Inport
  GnssConfig : Inport  Port=2
  fix_available : Inport  Port=3
  Disabled Output : Constant  Value=zeros(3,1)
  Is Failure : simulink/Logic and Bit Operations/Compare To Constant  relop===  const=3  OutDataTypeStr=boolean
  No Fix Output : Constant  Value=zeros(3,1)
  Select Enabled : Switch  Criteria=u2 > Threshold  Threshold=0.5  SaturateOnIntegerOverflow=off  InputSameDT=off
  Select Failure : Switch  Criteria=u2 > Threshold  Threshold=0.5  SaturateOnIntegerOverflow=off  InputSameDT=off
  Select Fix : Switch  Criteria=u2 > Threshold  Threshold=0.5  SaturateOnIntegerOverflow=off  InputSameDT=off
  Select GNSS Config : BusSelector  OutputSignals=enabled,mode_id,failure_v_I_m_s
  v_I_m_s : Outport
  wires:
  vNominal_I_m_s/1 -> Select Fix/1
  fix_available/1 -> Select Fix/2
  No Fix Output/1 -> Select Fix/3
  [FAIL_VALUE] -> Select Failure/1
  [IS_FAILURE] -> Select Failure/2
  Select Fix/1 -> Select Failure/3
  Select Failure/1 -> Select Enabled/1
  [ENABLED] -> Select Enabled/2
  Disabled Output/1 -> Select Enabled/3
  Select Enabled/1 -> v_I_m_s/1  "v_I_m_s"
  GnssConfig/1 -> Select GNSS Config/1
  Select GNSS Config/1 -> [ENABLED]  "<enabled>"
  Select GNSS Config/2 -> Is Failure/1  "<mode_id>"
  Is Failure/1 -> [IS_FAILURE]
  Select GNSS Config/3 -> [FAIL_VALUE]  "<failure_v_I_m_s>"

== system aocs_plant/Sensors/GNSS/PVT Error Model/Position Error RTN ==
  Gauss-Markov : Subsystem
  Ionosphere Bias : Constant  Value=[AOCS_SensorConfig.GNSS.radial_ionosphere_bias_m; 0; 0]
  Orbital Phase Sine : Sin  Frequency=AOCS_SensorConfig.GNSS.once_per_orbit_angular_rate_rad_s  Phase=AOCS_SensorConfig.GNSS.once_per_orbit_phase_rad  SampleTime=AOCS_SensorConfig.GNSS.sample_time_s
  Position Periodic Amplitude : Gain  Gain=AOCS_SensorConfig.GNSS.position_periodic_amplitude_RTN_m  Multiplication=Matrix(K*u)
  Sum Errors : Sum  Inputs=++++
  White Noise Std : Gain  Gain=diag(AOCS_SensorConfig.GNSS.position_white_noise_std_RTN_m)  Multiplication=Matrix(K*u)
  White Noise W : RandomNumber  Mean=zeros(3,1)  Variance=ones(3,1)  Seed=AOCS_SensorConfig.GNSS.position_white_noise_seed  SampleTime=AOCS_SensorConfig.GNSS.sample_time_s
  positionError_RTN_m : Outport
  wires:
  Orbital Phase Sine/1 -> Position Periodic Amplitude/1
  Ionosphere Bias/1 -> Sum Errors/1  "ionosphere_bias_RTN_m"
  Position Periodic Amplitude/1 -> Sum Errors/2  "periodic_position_RTN_m"
  Gauss-Markov/1(state) -> Sum Errors/3  "colored_position_RTN_m"
  White Noise W/1 -> White Noise Std/1
  White Noise Std/1 -> Sum Errors/4  "white_position_RTN_m"
  Sum Errors/1 -> positionError_RTN_m/1  "position_error_RTN_m"

== system aocs_plant/Sensors/GNSS/PVT Error Model/Velocity Error RTN ==
  Gauss-Markov : Subsystem
  Orbital Phase Sine : Sin  Frequency=AOCS_SensorConfig.GNSS.once_per_orbit_angular_rate_rad_s  Phase=AOCS_SensorConfig.GNSS.once_per_orbit_phase_rad  SampleTime=AOCS_SensorConfig.GNSS.sample_time_s
  Sum Errors : Sum  Inputs=+++
  Velocity Periodic Amplitude : Gain  Gain=AOCS_SensorConfig.GNSS.velocity_periodic_amplitude_RTN_m_s  Multiplication=Matrix(K*u)
  White Noise Std : Gain  Gain=diag(AOCS_SensorConfig.GNSS.velocity_white_noise_std_RTN_m_s)  Multiplication=Matrix(K*u)
  White Noise W : RandomNumber  Mean=zeros(3,1)  Variance=ones(3,1)  Seed=AOCS_SensorConfig.GNSS.velocity_white_noise_seed  SampleTime=AOCS_SensorConfig.GNSS.sample_time_s
  velocityError_RTN_m_s : Outport
  wires:
  Orbital Phase Sine/1 -> Velocity Periodic Amplitude/1
  Velocity Periodic Amplitude/1 -> Sum Errors/1  "periodic_velocity_RTN_m_s"
  Gauss-Markov/1(state) -> Sum Errors/2  "colored_velocity_RTN_m_s"
  White Noise W/1 -> White Noise Std/1
  White Noise Std/1 -> Sum Errors/3  "white_velocity_RTN_m_s"
  Sum Errors/1 -> velocityError_RTN_m_s/1  "velocity_error_RTN_m_s"

== system aocs_plant/Flight Dynamics/Orbit & Environment/Disturbance Torques/Aerodynamic Disturbance Path/Relative Wind ==
  OrbitState : Inport  OutDataTypeStr=Bus: OrbitStateBus
  AttitudeState : Inport  Port=2  OutDataTypeStr=Bus: AttitudeStateBus
  Atmosphere : Inport  Port=3  OutDataTypeStr=Bus: AtmosphereBus
  Relative Wind Products : MATLAB Function  TreatAsAtomicUnit=on
  Select Atmosphere : BusSelector  OutputSignals=v_atm_I_m_s,rho_kg_m3
  Select Attitude State : BusSelector  OutputSignals=DCM_be
  Select Orbit State : BusSelector  OutputSignals=v_I_m_s
  v_flow_B_m_s : Outport  OutDataTypeStr=double
  v_rel_norm_m_s : Outport  Port=2  OutDataTypeStr=double
  q_dyn_N_m2 : Outport  Port=3  OutDataTypeStr=double
  wires:
  Relative Wind Products/3(q_dyn_N_m2) -> q_dyn_N_m2/1
  Relative Wind Products/2(v_rel_norm_m_s) -> v_rel_norm_m_s/1
  Relative Wind Products/1(v_flow_B_m_s) -> v_flow_B_m_s/1
  Select Atmosphere/2 -> Relative Wind Products/4(rho_kg_m3)  "<rho_kg_m3>"
  Select Attitude State/1 -> Relative Wind Products/3(DCM_be)  "<DCM_be>"
  Select Atmosphere/1 -> Relative Wind Products/2(v_atm_I_m_s)  "<v_atm_I_m_s>"
  Select Orbit State/1 -> Relative Wind Products/1(v_I_m_s)  "<v_I_m_s>"
  Atmosphere/1 -> Select Atmosphere/1
  AttitudeState/1 -> Select Attitude State/1
  OrbitState/1 -> Select Orbit State/1
